simulink model "schemat_liniowy"  (R2018a)
settings: Solver=VariableStepAuto  StartTime=0.0  StopTime=10.0  RelTol=1e-3
values from neighbouring files (symbols this model uses):
  A1 = 4    [liniowy.m]    (also in nieliniowy.m)
  a1 = Aw1*sqrt((2*g)/h_max)    [liniowy.m]
  A2 = 4    [liniowy.m]    (also in nieliniowy.m)
  a2 = Aw2*sqrt((2*g)/h_max)    [liniowy.m]
  dfwe = 0.1*fwe_max    [liniowy.m]    (also in nieliniowy.m)
  fwe = 0.5*fwe_max    [liniowy.m]    (also in nieliniowy.m = 0*fwe_max)
  h10 = fwe/a1    [liniowy.m]    (also in nieliniowy.m = (fwe^2)/((Aw1^2)*2*g))
  h20 = fwe/a2    [liniowy.m]    (also in nieliniowy.m = ((Aw1^2)*h10)/(Aw2^2))
settings Model: Creator=margr  LastModifiedBy=margr

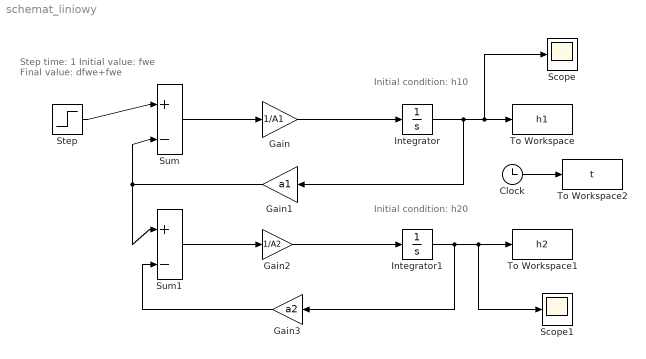
== system schemat_liniowy ==
  note: Initial condition: h20
  note: Initial condition: h10
  note: Step time: 1
      | Initial value: fwe
      | Final value: dfwe+fwe
  Clock : Clock
  Gain : Gain  Gain=1/A1
  Gain1 : Gain  Gain=a1
  Gain2 : Gain  Gain=1/A2
  Gain3 : Gain  Gain=a2
  Integrator : Integrator  InitialCondition=h10
  Integrator1 : Integrator  InitialCondition=h20
  Scope : Scope
  Scope1 : Scope
  Step : Step  Before=fwe  After=dfwe+fwe  SampleTime=0
  Sum : Sum  Inputs=|+-
  Sum1 : Sum  Inputs=|+-
  To Workspace : ToWorkspace  VariableName=h1  SampleTime=-1
  To Workspace1 : ToWorkspace  VariableName=h2  SampleTime=-1
  To Workspace2 : ToWorkspace  VariableName=t  SaveFormat=Timeseries  SampleTime=-1
  wires:
  Step/1 -> Sum/1
  Sum/1 -> Gain/1
  Gain/1 -> Integrator/1
  Integrator/1 -> Gain1/1, Scope/1, To Workspace/1
  Gain1/1 -> Sum1/1, Sum/2
  Sum1/1 -> Gain2/1
  Gain2/1 -> Integrator1/1
  Integrator1/1 -> Gain3/1, Scope1/1, To Workspace1/1
  Gain3/1 -> Sum1/2
  Clock/1 -> To Workspace2/1
